simulink model "commLink"  (R2022b)
settings: Solver=VariableStepAuto  StartTime=0.0  StopTime=10.0  RelTol=1e-3
undefined symbols (not defined in the file or in its folder): Data, Preamble
libraries: hdlsllib x5, commdigbbndam3 x1
settings Model: Creator=Ceribro  LastModifiedBy=Ceribro

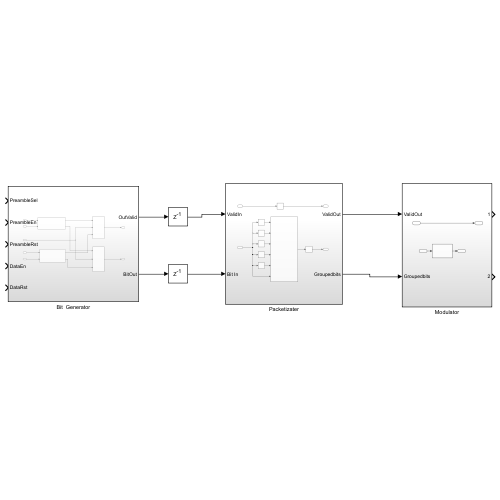
[thumbnail: Simulink's stored preview of the top-level diagram]
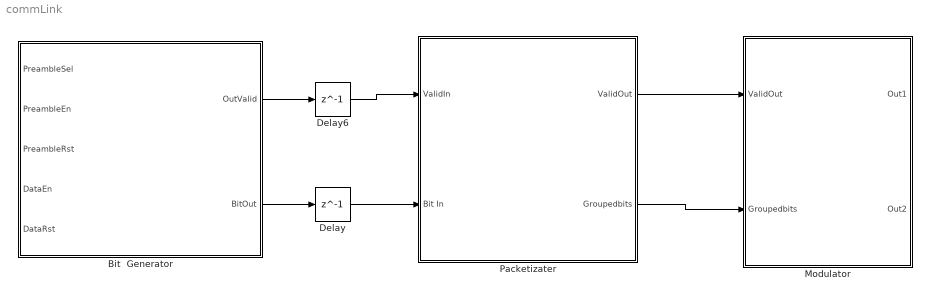
== system commLink ==
  Bit  Generator : Subsystem
  Delay : Delay  DelayLength=1  InitialCondition=0
  Delay6 : Delay  DelayLength=1  InitialCondition=0
  Modulator : Subsystem
  Packetizater : Subsystem
  wires:
  Bit  Generator/2(BitOut) -> Delay/1
  Delay/1 -> Packetizater/2(Bit In)
  Bit  Generator/1(OutValid) -> Delay6/1
  Delay6/1 -> Packetizater/1(ValidIn)
  Packetizater/1(ValidOut) -> Modulator/1(ValidOut)
  Packetizater/2(Groupedbits) -> Modulator/2(Groupedbits)

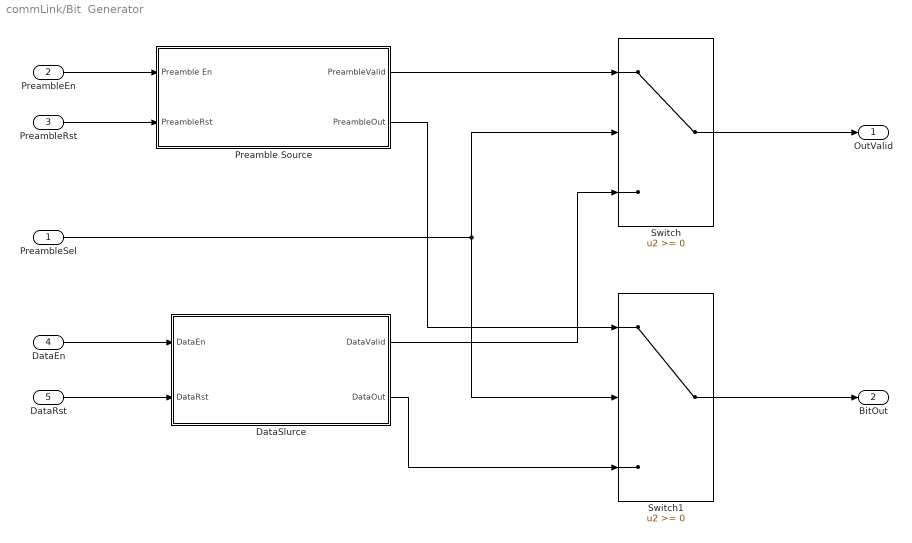
== system commLink/Bit  Generator ==
  PreambleSel : Inport
  PreambleEn : Inport  Port=2
  PreambleRst : Inport  Port=3
  DataEn : Inport  Port=4
  DataRst : Inport  Port=5
  DataSlurce : Subsystem
  Preamble Source : Subsystem
  Switch : Switch  SaturateOnIntegerOverflow=off  InputSameDT=off
  Switch1 : Switch  SaturateOnIntegerOverflow=off  InputSameDT=off
  OutValid : Outport
  BitOut : Outport  Port=2
  wires:
  PreambleEn/1 -> Preamble Source/1(Preamble En)
  Preamble Source/1(PreambleValid) -> Switch/1
  DataSlurce/1(DataValid) -> Switch/3
  PreambleRst/1 -> Preamble Source/2(PreambleRst)
  DataEn/1 -> DataSlurce/1(DataEn)
  PreambleSel/1 -> Switch1/2, Switch/2
  Preamble Source/2(PreambleOut) -> Switch1/1
  DataRst/1 -> DataSlurce/2(DataRst)
  DataSlurce/2(DataOut) -> Switch1/3
  Switch1/1 -> BitOut/1
  Switch/1 -> OutValid/1

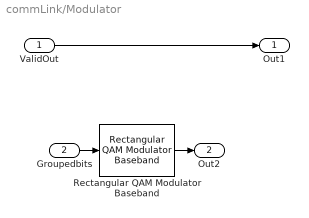
== system commLink/Modulator ==
  ValidOut : Inport
  Groupedbits : Inport  Port=2
  Rectangular QAM Modulator Baseband : commdigbbndam3/Rectangular QAM Modulator Baseband  M=64  InType=Integer  Enc=Gray  Mapping=[0:15]  PowType=Min. distance between symbols  MinDist=2  AvgPow=1  PeakPow=1  Ph=0  outDtype=double  outWordLen=16  outUDDataType=sfix(16)  outFracLenMode=Best precision  outFracLen=15  outDataTypeStr=double  outLastDataTypeStr=double
      settings: LibrarySourceBlock=|
      | commhdldigbbndam/Rectangular QAM
      | Modulator
      | Baseband
  Out1 : Outport
  Out2 : Outport  Port=2
  wires:
  ValidOut/1 -> Out1/1
  Groupedbits/1 -> Rectangular QAM Modulator Baseband/1
  Rectangular QAM Modulator Baseband/1 -> Out2/1

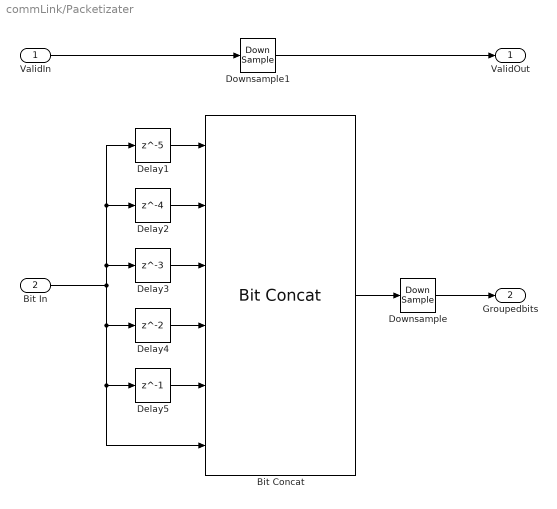
== system commLink/Packetizater ==
  ValidIn : Inport
  Bit In : Inport  Port=2
  Bit Concat : hdlsllib/Logic and Bit Operations/Bit Concat  numInputs=6
  Delay1 : Delay  DelayLength=5  InitialCondition=0
  Delay2 : Delay  DelayLength=4  InitialCondition=0
  Delay3 : Delay  DelayLength=3  InitialCondition=0
  Delay4 : Delay  InitialCondition=0
  Delay5 : Delay  DelayLength=1  InitialCondition=0
  Downsample : DownSample  N=6  phase=2  RateOptions=Allow multirate processing
  Downsample1 : DownSample  N=6  phase=2  RateOptions=Allow multirate processing
  ValidOut : Outport
  Groupedbits : Outport  Port=2
  wires:
  Bit In/1 -> Delay4/1, Bit Concat/6, Delay5/1, Delay3/1, Delay2/1, Delay1/1
  Delay1/1 -> Bit Concat/1
  ValidIn/1 -> Downsample1/1
  Bit Concat/1 -> Downsample/1
  Delay5/1 -> Bit Concat/5
  Delay4/1 -> Bit Concat/4
  Downsample/1 -> Groupedbits/1
  Delay3/1 -> Bit Concat/3
  Delay2/1 -> Bit Concat/2
  Downsample1/1 -> ValidOut/1

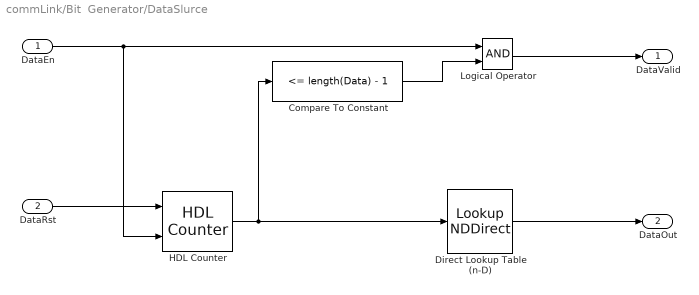
== system commLink/Bit  Generator/DataSlurce ==
  DataEn : Inport
  DataRst : Inport  Port=2
  Compare To Constant : hdlsllib/Logic and Bit Operations/Compare To Constant  relop=<=  const=length(Data) - 1  OutDataTypeStr=boolean
  Direct Lookup Table (n-D) : LookupNDDirect  NumberOfTableDimensions=1  Table=[Preamble ]  DiagnosticForOutOfRangeInput=Error
  HDL Counter : hdlsllib/Sources/HDL Counter  CountType=Count limited  CountInit=0  CountStep=1  CountMax=length(Data) - 1  CountFromType=Initial value  CountFrom=0  CountResetPort=on  CountLoadPort=off  CountEnbPort=on  CountDirPort=off  CountHitOutputPort=off  CountDataType=Unsigned  CountWordLen=8  CountFracLen=0  CountSampTime=1
  Logical Operator : Logic  AllPortsSameDT=off  OutDataTypeStr=boolean
  DataValid : Outport
  DataOut : Outport  Port=2
  wires:
  HDL Counter/1 -> Compare To Constant/1, Direct Lookup Table (n-D)/1
  Compare To Constant/1 -> Logical Operator/2
  Logical Operator/1 -> DataValid/1
  DataRst/1 -> HDL Counter/1
  Direct Lookup Table (n-D)/1 -> DataOut/1
  DataEn/1 -> HDL Counter/2, Logical Operator/1

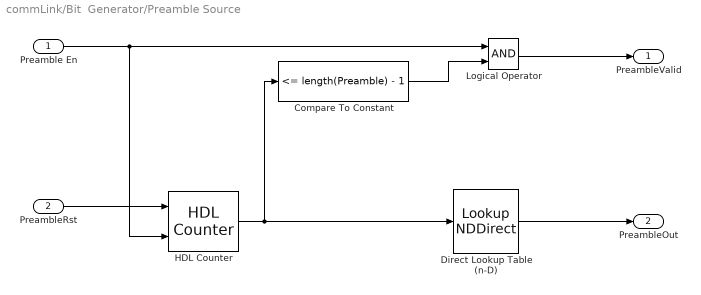
== system commLink/Bit  Generator/Preamble Source ==
  Preamble En : Inport
  PreambleRst : Inport  Port=2
  Compare To Constant : hdlsllib/Logic and Bit Operations/Compare To Constant  relop=<=  const=length(Preamble) - 1  OutDataTypeStr=boolean
  Direct Lookup Table (n-D) : LookupNDDirect  NumberOfTableDimensions=1  Table=[Preamble ]  DiagnosticForOutOfRangeInput=Error
  HDL Counter : hdlsllib/Sources/HDL Counter  CountType=Count limited  CountInit=0  CountStep=1  CountMax=length(Preamble) - 1  CountFromType=Initial value  CountFrom=0  CountResetPort=on  CountLoadPort=off  CountEnbPort=on  CountDirPort=off  CountHitOutputPort=off  CountDataType=Unsigned  CountWordLen=8  CountFracLen=0  CountSampTime=1
  Logical Operator : Logic  AllPortsSameDT=off  OutDataTypeStr=boolean
  PreambleValid : Outport
  PreambleOut : Outport  Port=2
  wires:
  Direct Lookup Table (n-D)/1 -> PreambleOut/1
  HDL Counter/1 -> Compare To Constant/1, Direct Lookup Table (n-D)/1
  Preamble En/1 -> HDL Counter/2, Logical Operator/1
  PreambleRst/1 -> HDL Counter/1
  Logical Operator/1 -> PreambleValid/1
  Compare To Constant/1 -> Logical Operator/2
